simulink model "ABS_contDyn_model"  (R2024b)
settings: Solver=VariableStepAuto  StartTime=0.0  StopTime=tf  MaxStep=1e-3  RelTol=1e-3  EnableMultiTasking=on
values from neighbouring files (symbols this model uses):
  dt = 1e-3    (= 0.001)    [mainABS.m]
  init_speed = 100    [mainABS.m]
  omega_act = 70    [mainABS.m]
  tau_delay = 10e-3    (= 0.01)    [mainABS.m]
  Tb_max = 1500    [mainABS.m]
undefined symbols (not defined in the file or in its folder): auxdata, rnn, smc
libraries: simulink x2
settings Model: Creator=luca  LastModifiedBy=piyus
settings SolverCC: AlgebraicLoopSolver=TrustRegion
settings DataIOCC: LimitDataPoints=on  ReturnWorkspaceOutputs=off
settings OptimizationCC: ReuseModelBlockBuffer=off  LifeSpan=inf
settings DebuggingCC: UnconnectedInputMsg=warning  UnconnectedOutputMsg=warning  UnconnectedLineMsg=warning  AllowSymbolicDim=off  SFUnexpectedBacktrackingDiag=warning  SFNoUnconditionalDefaultTransitionDiag=warning  SFExecutionAtInitializationDiag=none  ArithmeticOperatorsInVariantConditions=warning
settings ModelReferenceCC: EnableRefExpFcnMdlSchedulingChecks=on  PropagateSignalLabelsOutOfModel=off
settings SFSimCC: SimUseLocalCustomCode=off  CustomCodeUndefinedFunction=UseInterfaceOnly
settings RTWCC: RTWUseLocalCustomCode=off  GPUComputeCapability=3.5
settings CodeAppCC: StateflowObjectComments=on
settings GRTTargetCC: TargetLangStandard=C89/C90 (ANSI)
settings ConfigComp: CovMetricSettings=dw  CovSaveCumulativeToWorkspaceVar=on  CovSaveSingleToWorkspaceVar=on  CovExternalEMLEnable=off

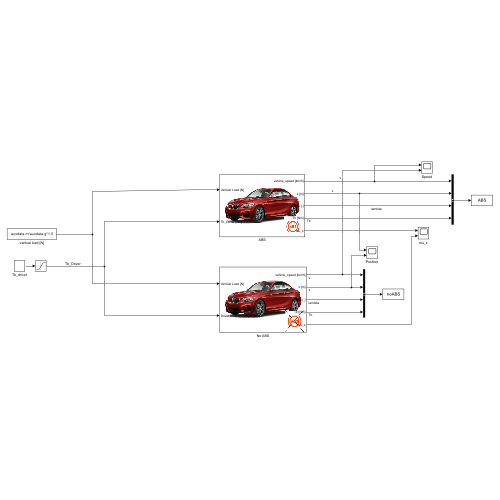
[thumbnail: Simulink's stored preview of the top-level diagram]
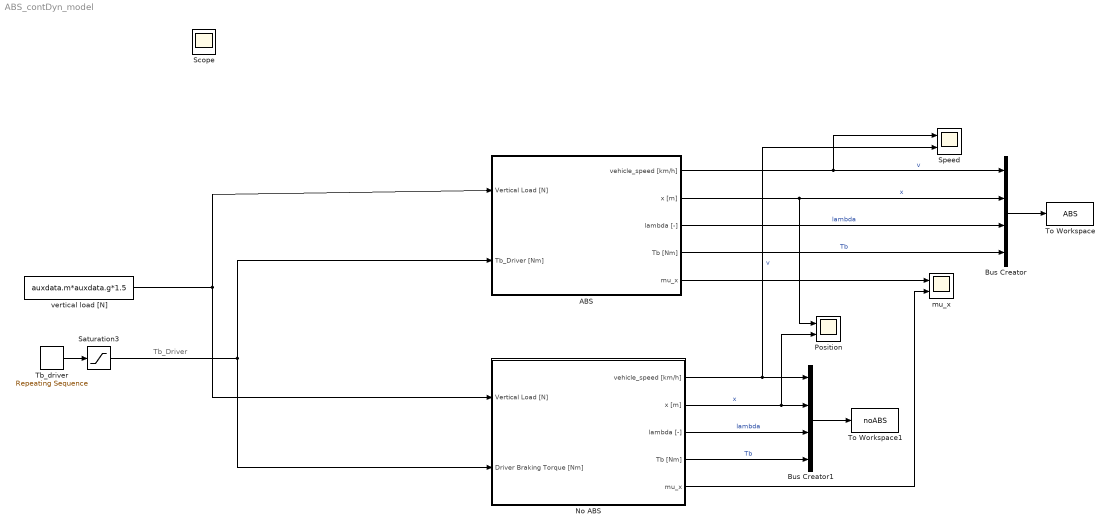
== system ABS_contDyn_model ==
  note: Tb_Driver
  ABS : Subsystem
      mask Display: image('figures/ABScar_on.png');
  Bus Creator : BusCreator  Inputs=4
  Bus Creator1 : BusCreator  Inputs=4
  No ABS : Subsystem
      mask Display: image('figures/ABS_off.png');
  Position : Scope  NumInputPorts=2
  Saturation3 : Saturate  UpperLimit=Tb_max  LowerLimit=0
  Speed : Scope  NumInputPorts=2
  Tb_driver : simulink/Sources/Repeating Sequence  rep_seq_t=time_manoeuvre  rep_seq_y=output_manoeuvre
  To Workspace : ToWorkspace  VariableName=ABS  SaveFormat=Timeseries  SampleTime=-1
  To Workspace1 : ToWorkspace  VariableName=noABS  SaveFormat=Timeseries  SampleTime=-1
  mu_x : Scope  NumInputPorts=2
  vertical load [N] : Constant  Value=auxdata.m*auxdata.g*1.5
  Scope : Scope
  wires:
  vertical load [N]/1 -> No ABS/1(Vertical Load [N]), ABS/1(Vertical Load [N])
  Saturation3/1 -> No ABS/2(Driver Braking Torque [Nm]), ABS/2(Tb_Driver [Nm])
  No ABS/1(" vehicle_speed [km/h]") -> Speed/2, Bus Creator1/1  "v"
  No ABS/2(x [m]) -> Position/2, Bus Creator1/2  "x"
  ABS/1(vehicle_speed [km/h]) -> Bus Creator/1, Speed/1  "v"
  ABS/2(x [m]) -> Bus Creator/2, Position/1  "x"
  Bus Creator/1 -> To Workspace/1
  ABS/3(lambda [-]) -> Bus Creator/3  "lambda"
  ABS/4(Tb [Nm]) -> Bus Creator/4  "Tb"
  Bus Creator1/1 -> To Workspace1/1
  No ABS/3(lambda [-]) -> Bus Creator1/3  "lambda"
  No ABS/4(Tb [Nm]) -> Bus Creator1/4  "Tb"
  Tb_driver/1 -> Saturation3/1
  ABS/5(mu_x) -> mu_x/1
  No ABS/5(" mu_x") -> mu_x/2

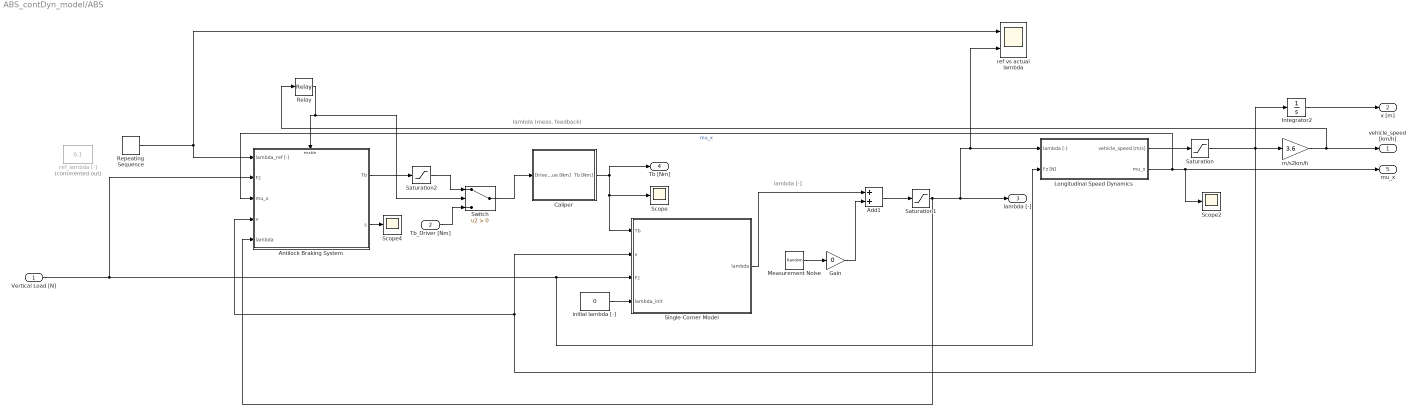
== system ABS_contDyn_model/ABS ==
  note: lambda [-]
  note: lambda (meas. feedback)
  Vertical Load [N] : Inport
  Tb_Driver [Nm] : Inport  Port=2
  Add1 : Sum
  Antilock Braking System : Subsystem
      mask Display: image('figures/ABS_on.png');
  Caliper : Subsystem
  Gain : Gain  Gain=0
  Integrator2 : Integrator
  Longitudinal Speed Dynamics : Subsystem
  Measurement Noise : RandomNumber  Variance=2e-5  SampleTime=0.001
  Relay : Relay  OnSwitchValue=6  OffSwitchValue=4
  Repeating Sequence : simulink/Sources/Repeating Sequence  rep_seq_t=time_manoeuvre  rep_seq_y=lambda_required
  Saturation : Saturate  UpperLimit=100  LowerLimit=1e-3
  Saturation1 : Saturate  UpperLimit=1  LowerLimit=0
  Saturation2 : Saturate  UpperLimit=1500  LowerLimit=0
  Scope : Scope
  Scope2 : Scope
  Scope4 : Scope
  Single-Corner Model : Subsystem
      mask Display:
      | image('figures/caliper_img.jpeg');
      | color('red');
      | port_label('output',1,'lambda');
      | port_label('input',1,'Tb');
      | port_label('input',2,'v');
      | port_label('input',3,'Fz');
      | port_label('input',4,'lambda_init');
  Switch : Switch  Criteria=u2 > Threshold  SaturateOnIntegerOverflow=off  InputSameDT=off
  initial lambda [-] : Constant  Value=0
  m/s2km/h : Gain  Gain=3.6
  ref vs actual lambda : Scope  NumInputPorts=2
  ref_lambda [-] : Constant  Commented=on  Value=0.1
  vehicle_speed [km/h] : Outport
  x [m] : Outport  Port=2
  lambda [-] : Outport  Port=3
  Tb [Nm] : Outport  Port=4
  mu_x : Outport  Port=5
  wires:
  Integrator2/1 -> x [m]/1
  Longitudinal Speed Dynamics/1(vehicle_speed [m/s]) -> Saturation/1
  Caliper/1(Tb [Nm]) -> Scope/1, Single-Corner Model/1(Tb), Tb [Nm]/1
  Saturation1/1 -> lambda [-]/1, ref vs actual lambda/2, Longitudinal Speed Dynamics/1(lambda [-]), Antilock Braking System/5(lambda)
  Gain/1 -> Add1/2
  Single-Corner Model/1(lambda) -> Add1/1
  Saturation/1 -> Single-Corner Model/2(v), Antilock Braking System/4(v), Integrator2/1, m/s2km/h/1
  Add1/1 -> Saturation1/1
  Measurement Noise/1 -> Gain/1
  Vertical Load [N]/1 -> Antilock Braking System/2(Fz), Single-Corner Model/3(Fz), Longitudinal Speed Dynamics/2(Fz [N])
  initial lambda [-]/1 -> Single-Corner Model/4(lambda_init)
  Longitudinal Speed Dynamics/2(mu_x) -> Antilock Braking System/3(mu_x), Scope2/1, mu_x/1  "mu_x"
  Antilock Braking System/2(s) -> Scope4/1
  Repeating Sequence/1 -> Antilock Braking System/1(lambda_ref [-]), ref vs actual lambda/1
  m/s2km/h/1 -> Relay/1, vehicle_speed [km/h]/1
  Antilock Braking System/1(Tb) -> Saturation2/1
  Relay/1 -> Switch/2, Antilock Braking System/Enable
  Saturation2/1 -> Switch/1
  Tb_Driver [Nm]/1 -> Switch/3
  Switch/1 -> Caliper/1(Driver Braking  Torque [Nm])

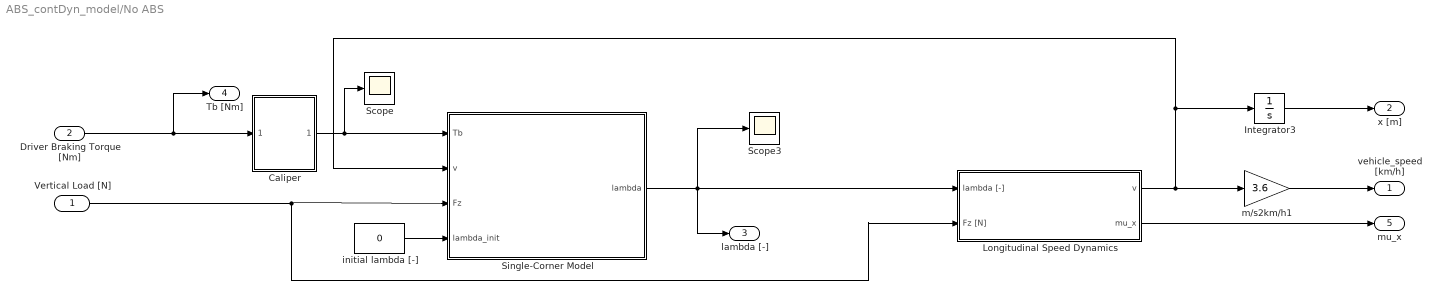
== system ABS_contDyn_model/No ABS ==
  Vertical Load [N] : Inport
  Driver Braking Torque [Nm] : Inport  Port=2
  Caliper : Subsystem
  Integrator3 : Integrator
  Longitudinal Speed Dynamics : Subsystem
  Scope : Scope
  Scope3 : Scope
  Single-Corner Model : Subsystem
      mask Display:
      | image('figures/caliper_img.jpeg');
      | color('red');
      | port_label('output',1,'lambda');
      | port_label('input',1,'Tb');
      | port_label('input',2,'v');
      | port_label('input',3,'Fz');
      | port_label('input',4,'lambda_init');
  initial lambda [-] : Constant  Value=0
  m/s2km/h1 : Gain  Gain=3.6
  " vehicle_speed [km/h]" : Outport
  x [m] : Outport  Port=2
  lambda [-] : Outport  Port=3
  Tb [Nm] : Outport  Port=4
  " mu_x" : Outport  Port=5
  wires:
  Single-Corner Model/1(lambda) -> lambda [-]/1, Longitudinal Speed Dynamics/1(lambda [-]), Scope3/1
  Vertical Load [N]/1 -> Longitudinal Speed Dynamics/2(Fz [N]), Single-Corner Model/3(Fz)
  Driver Braking Torque [Nm]/1 -> Tb [Nm]/1, Caliper/1(Driver Braking Torque [Nm])
  initial lambda [-]/1 -> Single-Corner Model/4(lambda_init)
  m/s2km/h1/1 -> " vehicle_speed [km/h]"/1
  Integrator3/1 -> x [m]/1
  Longitudinal Speed Dynamics/1(v) -> Integrator3/1, Single-Corner Model/2(v), m/s2km/h1/1
  Longitudinal Speed Dynamics/2(mu_x) -> " mu_x"/1
  Caliper/1(Tb [Nm]) -> Scope/1, Single-Corner Model/1(Tb)

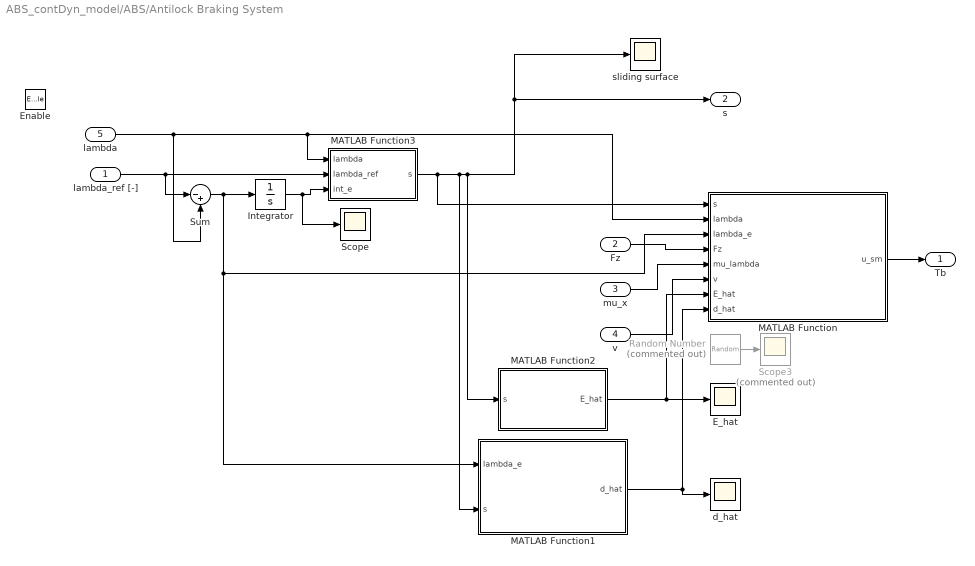
== system ABS_contDyn_model/ABS/Antilock Braking System ==
  lambda_ref [-] : Inport
  Fz : Inport  Port=2
  mu_x : Inport  Port=3
  v : Inport  Port=4
  lambda : Inport  Port=5
  Enable : EnablePort
  E_hat : Scope
  Integrator : Integrator
  MATLAB Function : MATLAB Function  TreatAsAtomicUnit=on
  MATLAB Function1 : MATLAB Function  TreatAsAtomicUnit=on  SystemSampleTime=0.001
  MATLAB Function2 : MATLAB Function  TreatAsAtomicUnit=on
  MATLAB Function3 : MATLAB Function  TreatAsAtomicUnit=on
  Random Number : RandomNumber  Commented=on  SampleTime=0.001
  Scope : Scope
  Scope3 : Scope  Commented=on
  Sum : Sum  Inputs=|-+
  d_hat : Scope
  sliding surface : Scope
  Tb : Outport
  s : Outport  Port=2
  wires:
  lambda/1 -> MATLAB Function/2(lambda), MATLAB Function3/1(lambda), Sum/2
  lambda_ref [-]/1 -> MATLAB Function3/2(lambda_ref), Sum/1
  Integrator/1 -> Scope/1, MATLAB Function3/3(int_e)
  Sum/1 -> MATLAB Function1/1(lambda_e), MATLAB Function/3(lambda_e), Integrator/1
  MATLAB Function3/1(s) -> MATLAB Function2/1(s), s/1, sliding surface/1, MATLAB Function1/2(s), MATLAB Function/1(s)
  Fz/1 -> MATLAB Function/4(Fz)
  mu_x/1 -> MATLAB Function/5(mu_lambda)
  v/1 -> MATLAB Function/6(v)
  MATLAB Function2/1(E_hat) -> E_hat/1, MATLAB Function/7(E_hat)
  MATLAB Function1/1(d_hat) -> MATLAB Function/8(d_hat), d_hat/1
  MATLAB Function/1(u_sm) -> Tb/1
  Random Number/1 -> Scope3/1

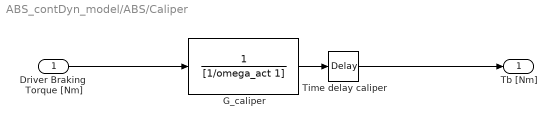
== system ABS_contDyn_model/ABS/Caliper ==
  Driver Braking  Torque [Nm] : Inport
  G_caliper : TransferFcn  Numerator=1  Denominator=[1/omega_act 1]
  Time delay caliper : TransportDelay  DelayTime=tau_delay
  Tb [Nm] : Outport
  wires:
  Time delay caliper/1 -> Tb [Nm]/1
  Driver Braking  Torque [Nm]/1 -> G_caliper/1
  G_caliper/1 -> Time delay caliper/1

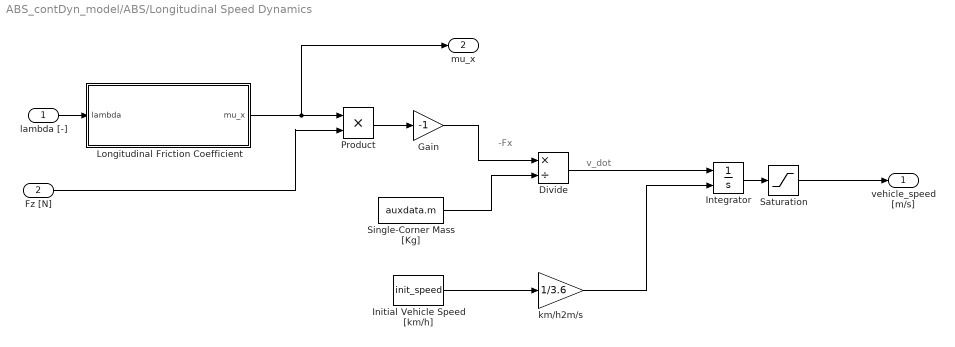
== system ABS_contDyn_model/ABS/Longitudinal Speed Dynamics ==
  note: -Fx
  note: v_dot
  lambda [-] : Inport
  Fz [N] : Inport  Port=2
  Divide : Product  Inputs=*/
  Gain : Gain  Gain=-1
  Initial Vehicle Speed [km/h] : Constant  Value=init_speed
  Integrator : Integrator  InitialConditionSource=external
  Longitudinal Friction Coefficient : MATLAB Function  TreatAsAtomicUnit=on
  Product : Product
  Saturation : Saturate  UpperLimit=100  LowerLimit=0
  Single-Corner Mass [Kg] : Constant  Value=auxdata.m
  km/h2m/s : Gain  Gain=1/3.6
  vehicle_speed [m/s] : Outport
  mu_x : Outport  Port=2
  wires:
  Single-Corner Mass [Kg]/1 -> Divide/2
  Divide/1 -> Integrator/1
  km/h2m/s/1 -> Integrator/2
  Initial Vehicle Speed [km/h]/1 -> km/h2m/s/1
  Product/1 -> Gain/1
  Gain/1 -> Divide/1
  Saturation/1 -> vehicle_speed [m/s]/1
  Integrator/1 -> Saturation/1
  Longitudinal Friction Coefficient/1(mu_x) -> mu_x/1, Product/1
  Fz [N]/1 -> Product/2
  lambda [-]/1 -> Longitudinal Friction Coefficient/1(lambda)

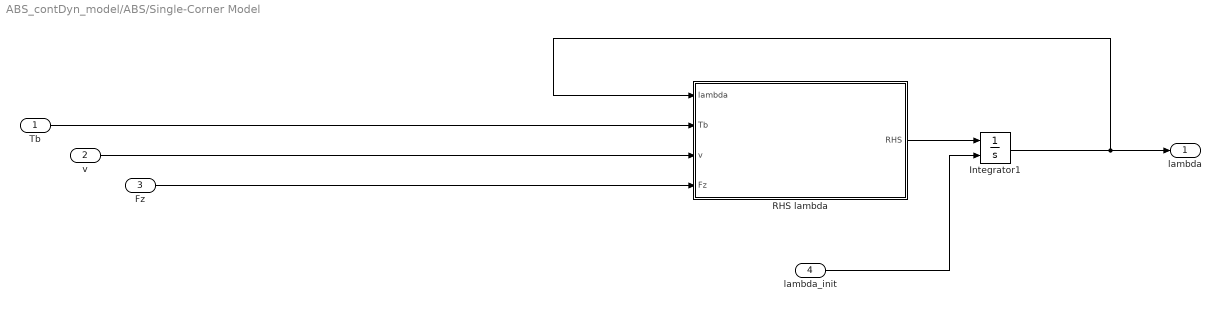
== system ABS_contDyn_model/ABS/Single-Corner Model ==
  Tb : Inport
  v : Inport  Port=2
  Fz : Inport  Port=3
  lambda_init : Inport  Port=4
  Integrator1 : Integrator  InitialConditionSource=external  LimitOutput=on  UpperSaturationLimit=1  LowerSaturationLimit=0
  RHS lambda : MATLAB Function  TreatAsAtomicUnit=on
  lambda : Outport
  wires:
  lambda_init/1 -> Integrator1/2
  RHS lambda/1(RHS) -> Integrator1/1
  v/1 -> RHS lambda/3(v)
  Fz/1 -> RHS lambda/4(Fz)
  Integrator1/1 -> RHS lambda/1(lambda), lambda/1
  Tb/1 -> RHS lambda/2(Tb)

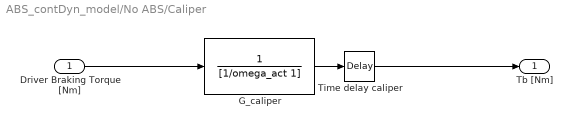
== system ABS_contDyn_model/No ABS/Caliper ==
  Driver Braking Torque [Nm] : Inport
  G_caliper : TransferFcn  Numerator=1  Denominator=[1/omega_act 1]
  Time delay caliper : TransportDelay  DelayTime=tau_delay
  Tb [Nm] : Outport
  wires:
  Time delay caliper/1 -> Tb [Nm]/1
  Driver Braking Torque [Nm]/1 -> G_caliper/1
  G_caliper/1 -> Time delay caliper/1

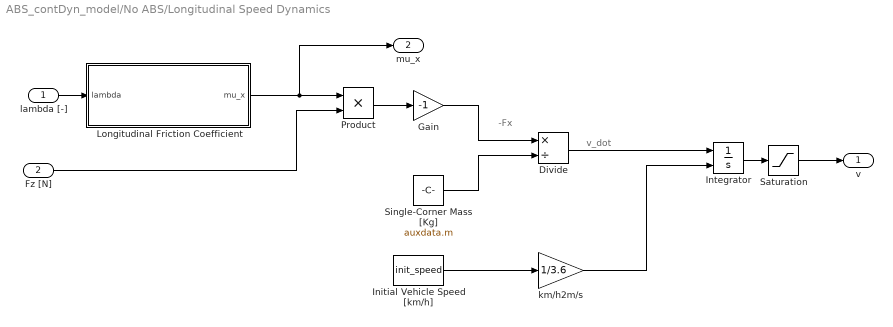
== system ABS_contDyn_model/No ABS/Longitudinal Speed Dynamics ==
  note: -Fx
  note: v_dot
  lambda [-] : Inport
  Fz [N] : Inport  Port=2
  Divide : Product  Inputs=*/
  Gain : Gain  Gain=-1
  Initial Vehicle Speed [km/h] : Constant  Value=init_speed
  Integrator : Integrator  InitialConditionSource=external
  Longitudinal Friction Coefficient : MATLAB Function  TreatAsAtomicUnit=on
  Product : Product
  Saturation : Saturate  UpperLimit=100  LowerLimit=1e-3
  Single-Corner Mass [Kg] : Constant  Value=auxdata.m
  km/h2m/s : Gain  Gain=1/3.6
  v : Outport
  mu_x : Outport  Port=2
  wires:
  Single-Corner Mass [Kg]/1 -> Divide/2
  Divide/1 -> Integrator/1
  km/h2m/s/1 -> Integrator/2
  Initial Vehicle Speed [km/h]/1 -> km/h2m/s/1
  Product/1 -> Gain/1
  Gain/1 -> Divide/1
  Saturation/1 -> v/1
  Integrator/1 -> Saturation/1
  Longitudinal Friction Coefficient/1(mu_x) -> mu_x/1, Product/1
  Fz [N]/1 -> Product/2
  lambda [-]/1 -> Longitudinal Friction Coefficient/1(lambda)

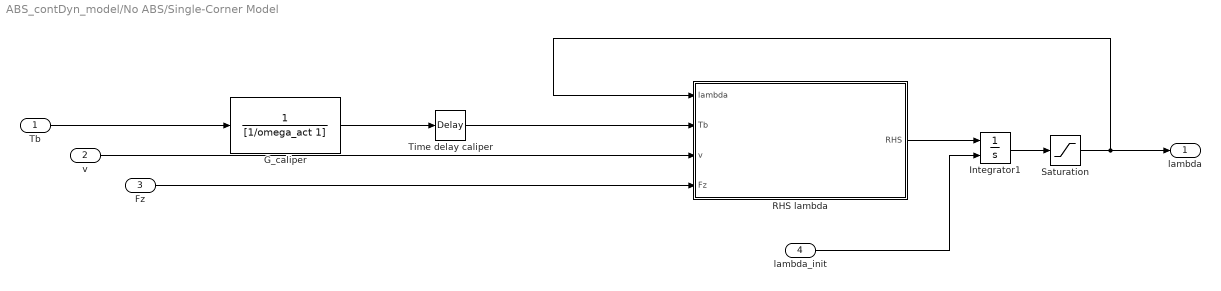
== system ABS_contDyn_model/No ABS/Single-Corner Model ==
  Tb : Inport
  v : Inport  Port=2
  Fz : Inport  Port=3
  lambda_init : Inport  Port=4
  G_caliper : TransferFcn  Numerator=1  Denominator=[1/omega_act 1]
  Integrator1 : Integrator  InitialConditionSource=external
  RHS lambda : MATLAB Function  TreatAsAtomicUnit=on
  Saturation : Saturate  UpperLimit=0.99  LowerLimit=0
  Time delay caliper : TransportDelay  DelayTime=tau_delay
  lambda : Outport
  wires:
  lambda_init/1 -> Integrator1/2
  RHS lambda/1(RHS) -> Integrator1/1
  v/1 -> RHS lambda/3(v)
  Fz/1 -> RHS lambda/4(Fz)
  Integrator1/1 -> Saturation/1
  G_caliper/1 -> Time delay caliper/1
  Time delay caliper/1 -> RHS lambda/2(Tb)
  Tb/1 -> G_caliper/1
  Saturation/1 -> RHS lambda/1(lambda), lambda/1

== matlab function ABS_contDyn_model/ABS/Antilock Braking System/MATLAB Function ==
  data: s input; lambda input; lambda_e input; Fz input; mu_lambda input; v input; u_sm output; auxdata parameter; smc parameter; E_hat input; d_hat input
function u_sm = controlLaw(s, lambda, lambda_e, Fz, mu_lambda, v, auxdata, smc, E_hat, d_hat)

  theta_nominal = 0;

  Bv_nominal   = 1.5; 
  Bw_nominal   = 4;

  N_v_nominal = auxdata.m * auxdata.g * cos(theta_nominal);
  F_theta_nominal = auxdata.m * auxdata.g * sin(theta_nominal);
  F_t = N_v_nominal * mu_lambda;
  T_t = auxdata.r_w * F_t;
  w_w = (1 - lambda) * v / auxdata.r_w;
  w_v = v / auxdata.r_w;

  sat_s = s/smc.phi;
  if sat_s > 1
      sat_s = 1;
  elseif sat_s < 1
      sat_s = -1;
  end

  

  % compute nominal drift f_n and control gain g_n
  fn = (((F_t + Bv_nominal * auxdata.r_w * w_v + F_theta_nominal) * lambda)/(auxdata.m * auxdata.r_w * w_v)) - (((F_t + Bv_nominal * auxdata.r_w * w_v + F_theta_nominal)*auxdata.J - (Bw_nominal * w_w - T_t)*auxdata.m * auxdata.r_w)/(auxdata.m * auxdata.r_w * w_v * auxdata.J));
  %fn = -(1/v)*(((1 - lambda)/auxdata.m) + auxdata.r_w^2/auxdata.J) * Fz * mu_lambda;
  gn =  auxdata.r_w /(auxdata.J * v);

  %lambda_ref_dot = diff(lambda_ref,time);
  lambda_ref_dot = 0;

  % equivalent control (forces ṡ=0 if no disturbance)
  u_eq = ( -fn + lambda_ref_dot - smc.k1*lambda_e - d_hat) / gn;
  
  % robust (switching) term
  u_rb = - (E_hat/gn) * sat_s;

  % robust (switching) term without RNN
  %u_rb = - (smc.rho/gn) * sign(s);

  % total SMC torque command
  u_sm = u_eq + u_rb;
end

== matlab function ABS_contDyn_model/ABS/Longitudinal Speed Dynamics/Longitudinal Friction Coefficient ==
  data: lambda input; mu_x output; auxdata parameter
function mu_x = LongitudinalFrction(lambda,auxdata)
    
mu_x = burckhardt(lambda,auxdata.road_condition);

end

== matlab function ABS_contDyn_model/No ABS/Single-Corner Model/RHS lambda ==
  data: lambda input; RHS output; Tb input; v input; Fz input; auxdata parameter
function RHS = lambdaDyn( lambda, Tb, v, Fz, auxdata )
% Right hand side of the longitudinal slip dynamics

omega = (1 - lambda) * v / auxdata.r_w;

% Equilibrium manifold
%        /      (1 - lambda) * J \
% Psi = | r_w + ----------------  | * Fz * mu
%        \          r_w * m      /
Psi = (auxdata.r_w + ...
       auxdata.J / (auxdata.r_w * auxdata.m) * (1 - lambda)) * Fz * ...
       burckhardt( lambda, auxdata.road_condition );

if omega <= 0.1
    RHS = 0;
else
    RHS = -(1 - lambda) / (auxdata.J * omega) * (Psi - Tb);
end

end

== matlab function ABS_contDyn_model/ABS/Antilock Braking System/MATLAB Function1 ==
  settings: updateMethod=DISCRETE  sampleTime=0.001
  data: lambda_e input; rnn parameter; s input; d_hat output; dt parameter
function d_hat = rnn_uncertainity_observer(lambda_e, rnn, s, dt)

persistent initialised;
persistent alpha_hat v_hat w_hat r_hat theta_hat; %RNN parameters
num_neurons = 5;
num_inputs = 1;

% --- One-time Initialization ---
if isempty(initialised)
    % Initialize weights with small random values instead of zeros or ones
    % to ensure neurons learn different features.
    rng('shuffle'); % Seed the random number generator
    alpha_hat = 0.01 * randn(num_neurons, 1);
    
    % Spread the centers across the expected input range.
    % Adjust the range [-1, 1] based on the expected values of lambda_e.
    v_hat = linspace(-1.0, 1.0, num_neurons);
    
    % Initialize widths to small random positive values
    w_hat = 0.1 * rand(num_inputs, num_neurons) + 1; % e.g., values between 1 and 1.1
    
    % Initialize recurrent weights to small random values
    r_hat = 0.01 * randn(num_neurons, 1); 
    
    % Neuron activation outputs
    theta_hat = zeros(num_neurons, 1);
    
    initialised = true;
end

%if isempty(initialised)

%    alpha_hat = zeros(num_neurons, 1);
 %   v_hat     = zeros(num_inputs, num_neurons);
 %   w_hat     = ones(num_inputs, num_neurons); 
 %   r_hat     = zeros(num_neurons, 1); 
 %   theta_hat = zeros(num_neurons, 1);
    
 %   initialised = true;
% end

eta1 = rnn.eta1;
eta2 = rnn.eta2;
eta3 = rnn.eta3;
eta4 = rnn.eta4;

x = lambda_e;
num_neurons = length(alpha_hat);
theta_previous = theta_hat;

% Initialize derivative matrices for the adaptive laws
A = zeros(num_neurons, num_neurons * num_inputs);
B = zeros(num_neurons, num_neurons * num_inputs);
C = zeros(num_neurons, num_neurons);


for k = 1:num_neurons

    recurrent_term = theta_previous(k)*r_hat(k);
    net_k = (w_hat(:, k)'.^2 .* (x + recurrent_term - v_hat(:, k)).^2);
    theta_hat(k) = exp(-net_k);

    dv = -2 * w_hat(:, k).^2 .* (x + recurrent_term - v_hat(:, k));
    dw = 2 * w_hat(:, k).* (x + recurrent_term - v_hat(:, k)).^2;
    dr = 2 * w_hat(:, k).^2 .* (x + recurrent_term - v_hat(:, k)) * theta_previous(k);

    A(k, (k-1)*num_inputs+1:k*num_inputs) = -theta_hat(k) * dv;
    B(k, (k-1)*num_inputs+1:k*num_inputs) = -theta_hat(k) * dw;
    C(k, k)                               = -theta_hat(k) * dr;   

end
d_hat = alpha_hat' * theta_hat;
alpha_hat_dot = eta1 * s * theta_hat;
v_hat_dot = eta2 * s * A' * alpha_hat;
w_hat_dot = eta3 * s * B' * alpha_hat;
r_hat_dot = eta4 * s * C' * alpha_hat;

alpha_hat = alpha_hat + alpha_hat_dot * dt;
v_hat     = v_hat + reshape(v_hat_dot, [num_inputs, num_neurons]) * dt;
w_hat     = w_hat + reshape(w_hat_dot, [num_inputs, num_neurons]) * dt;
r_hat     = r_hat + r_hat_dot * dt;

end

== matlab function ABS_contDyn_model/No ABS/Longitudinal Speed Dynamics/Longitudinal Friction Coefficient ==
  data: lambda input; mu_x output; auxdata parameter
function mu_x = LongitudinalFrction( lambda, auxdata )
    
mu_x = burckhardt( lambda, auxdata.road_condition );

end

== matlab function ABS_contDyn_model/ABS/Antilock Braking System/MATLAB Function2 ==
  settings: updateMethod=DISCRETE  sampleTime=0.001
  data: E_hat output; rnn parameter; dt parameter; s input
function E_hat = bound_estimaor(rnn, dt, s)
    
persistent initialised E_hat_persistent;

if isempty(initialised)
    % Initialize E_hat to zero on the first run
    E_hat_persistent = 0;
    initialised = true;
end

eta5 = rnn.eta5;
sigma_E = 0.05;

E_hat_dot = eta5 * (abs(s)  - sigma_E * E_hat_persistent);

% E_hat_dot = eta5 * abs(s);
E_hat_persistent = E_hat_persistent + E_hat_dot*dt;

E_hat = max(E_hat_persistent, 0);

end

== matlab function ABS_contDyn_model/ABS/Single-Corner Model/RHS lambda ==
  data: lambda input; RHS output; Tb input; v input; Fz input; auxdata parameter
function RHS = lambdaDyn( lambda, Tb, v, Fz, auxdata )
% Right hand side of the longitudinal slip dynamics

omega = (1 - lambda) * v / auxdata.r_w;

% Equilibrium manifold
%        /      (1 - lambda) * J \
% Psi = | r_w + ----------------  | * Fz * mu
%        \          r_w * m      /
Psi = (auxdata.r_w + ...
       auxdata.J / (auxdata.r_w * auxdata.m) * (1 - lambda)) * Fz * ...
       burckhardt( lambda, auxdata.road_condition );


if omega <= 0.1
    RHS = 0;
else
    RHS = -(1 - lambda) / (auxdata.J * omega) * (Psi - Tb);
end

end

== matlab function ABS_contDyn_model/ABS/Antilock Braking System/MATLAB Function3 ==
  data: lambda input; s output; lambda_ref input; int_e input; smc parameter
function s = smc(lambda, lambda_ref, int_e, smc)

% sliding surface
lambda_e = lambda - lambda_ref;
s = lambda_e + smc.k1 * int_e;
